simulink subsystem "debounce"  (R2022b)
settings: Solver=VariableStepAuto  StartTime=0.0  StopTime=10.0  RelTol=1e-3
Description:
  | Copyright (c) 2023, Alexei Evsenin, evsenin@gmail.com
settings Model: Creator=evsenin  LastModifiedBy=evsenin
settings ModelReferenceCC: EnableRefExpFcnMdlSchedulingChecks=on

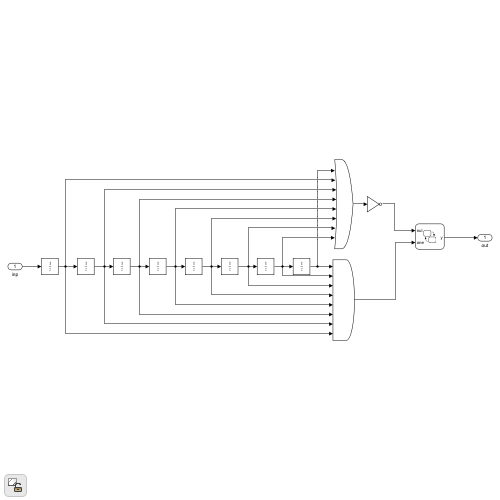
[thumbnail: Simulink's stored preview of the top-level diagram]
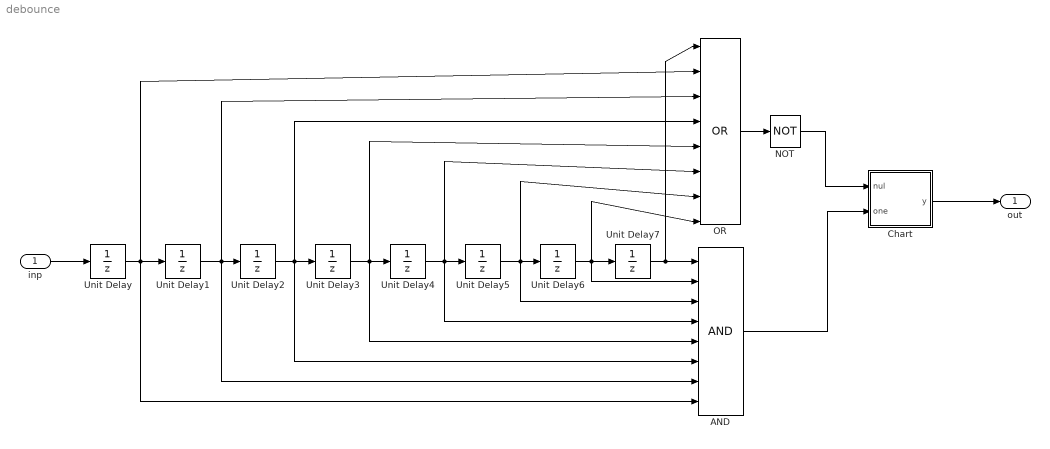
== system debounce ==
  inp : Inport
  AND : Logic  Inputs=8  IconShape=distinctive  AllPortsSameDT=off  OutDataTypeStr=boolean
  Chart : Stateflow chart  TreatAsAtomicUnit=on
  NOT : Logic  Operator=NOT  IconShape=distinctive  AllPortsSameDT=off  OutDataTypeStr=boolean
  OR : Logic  Operator=OR  Inputs=8  IconShape=distinctive  AllPortsSameDT=off  OutDataTypeStr=boolean
  Unit Delay{,1..7} (8 alike) : UnitDelay  SampleTime=-1  HasFrameUpgradeWarning=on
  out : Outport
  wires:
  Unit Delay/1 -> Unit Delay1/1, AND/8, OR/2
  Unit Delay1/1 -> Unit Delay2/1, AND/7, OR/3
  Unit Delay2/1 -> Unit Delay3/1, AND/6, OR/4
  Unit Delay3/1 -> Unit Delay4/1, AND/5, OR/5
  Unit Delay4/1 -> Unit Delay5/1, AND/4, OR/6
  Unit Delay5/1 -> Unit Delay6/1, AND/3, OR/7
  Unit Delay6/1 -> Unit Delay7/1, AND/2, OR/8
  inp/1 -> Unit Delay/1
  Unit Delay7/1 -> AND/1, OR/1
  AND/1 -> Chart/2(one)
  OR/1 -> NOT/1
  NOT/1 -> Chart/1(nul)
  Chart/1(y) -> out/1

== stateflow chart debounce/Chart ==
  settings: executeAtInitialization=1
  state ONE
    y = true;
  state RESET
    y = true;
  state NUL
    y = false;
  RESET -> ONE [order 1] : [one == true]
  (default) -> RESET
  NUL -> ONE : [one == true]
  ONE -> NUL : [nul == true]
  RESET -> NUL [order 2] : [nul == true]
  data: nul input; one input; y output
